simulink model "chap1_4"  (R2023b)
settings: Solver=ode45  StartTime=0.0  StopTime=5  RelTol=1e-3
settings Model: Creator=CorgiQvm  LastModifiedBy=CorgiQvm
settings DataIOCC: ReturnWorkspaceOutputs=off

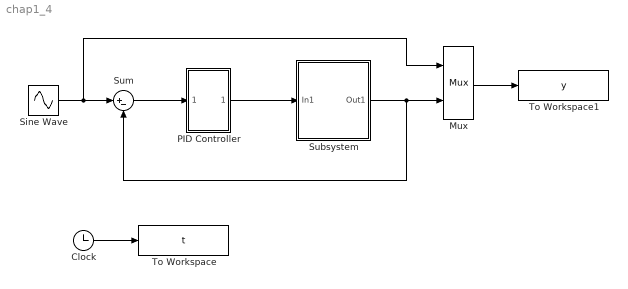
== system chap1_4 ==
  Clock : Clock
  Mux : Mux  Inputs=2
  PID Controller : Subsystem  mask{P=10, I=0, D=1}
      mask prompts: P "Proportional"; I "Integral"; D "Derivative"
      mask DialogControl ParameterGroupVar Prompt: 参数
      mask Display: disp('PID');
  Sine Wave : Sin  Amplitude=0.5  Frequency=1*2*pi  SampleTime=0
  Subsystem : Subsystem
  Sum : Sum  Inputs=|+-  InputSameDT=on  SaturateOnIntegerOverflow=on  OutDataTypeStr=Inherit: Same as first input
  To Workspace : ToWorkspace  VariableName=t  SampleTime=-1
  To Workspace1 : ToWorkspace  VariableName=y  SampleTime=-1
  wires:
  Clock/1 -> To Workspace/1
  Sine Wave/1 -> Mux/1, Sum/1
  Sum/1 -> PID Controller/1(In1)
  PID Controller/1(Out1) -> Subsystem/1(In1)
  Subsystem/1(Out1) -> Mux/2, Sum/2
  Mux/1 -> To Workspace1/1

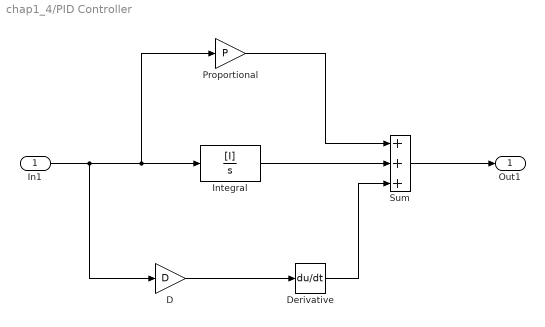
== system chap1_4/PID Controller ==
  In1 : Inport
  D : Gain  Gain=D  SaturateOnIntegerOverflow=on  OutDataTypeStr=Inherit: Same as input  ParamDataTypeStr=Inherit: Same as input
  Derivative : Derivative
  Integral : TransferFcn  Numerator=[I]  Denominator=[1 0]
  Proportional : Gain  Gain=P  SaturateOnIntegerOverflow=on  OutDataTypeStr=Inherit: Same as input  ParamDataTypeStr=Inherit: Same as input
  Sum : Sum  Inputs=+++  InputSameDT=on  SaturateOnIntegerOverflow=on  OutDataTypeStr=Inherit: Same as first input
  Out1 : Outport
  wires:
  D/1 -> Derivative/1
  Integral/1 -> Sum/2
  Proportional/1 -> Sum/1
  In1/1 -> D/1, Proportional/1, Integral/1
  Sum/1 -> Out1/1
  Derivative/1 -> Sum/3

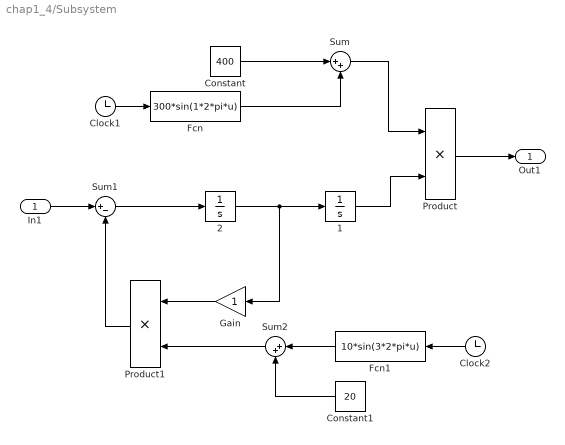
== system chap1_4/Subsystem ==
  In1 : Inport
  1 : Integrator
  2 : Integrator
  Clock1 : Clock
  Clock2 : Clock
  Constant : Constant  Value=400
  Constant1 : Constant  Value=20
  Fcn : Fcn  Expr=300*sin(1*2*pi*u)
  Fcn1 : Fcn  Expr=10*sin(3*2*pi*u)
  Gain : Gain  SaturateOnIntegerOverflow=on  OutDataTypeStr=Inherit: Same as input  ParamDataTypeStr=Inherit: Same as input
  Product : Product  InputSameDT=on  SaturateOnIntegerOverflow=on  OutDataTypeStr=Inherit: Same as first input
  Product1 : Product  InputSameDT=on  SaturateOnIntegerOverflow=on  OutDataTypeStr=Inherit: Same as first input
  Sum : Sum  Inputs=|++  InputSameDT=on  SaturateOnIntegerOverflow=on  OutDataTypeStr=Inherit: Same as first input
  Sum1 : Sum  Inputs=|+-  InputSameDT=on  SaturateOnIntegerOverflow=on  OutDataTypeStr=Inherit: Same as first input
  Sum2 : Sum  Inputs=|++  InputSameDT=on  SaturateOnIntegerOverflow=on  OutDataTypeStr=Inherit: Same as first input
  Out1 : Outport
  wires:
  Fcn/1 -> Sum/2
  Product/1 -> Out1/1
  Sum/1 -> Product/1
  Sum1/1 -> 2/1
  2/1 -> Gain/1, 1/1
  Fcn1/1 -> Sum2/1
  Constant1/1 -> Sum2/2
  Sum2/1 -> Product1/2
  Clock1/1 -> Fcn/1
  1/1 -> Product/2
  In1/1 -> Sum1/1
  Clock2/1 -> Fcn1/1
  Constant/1 -> Sum/1
  Gain/1 -> Product1/1
  Product1/1 -> Sum1/2
